simulink model "lab_5_task_2_simulink"  (R2025b)
settings: Solver=ode4  StartTime=0.0  StopTime=100  FixedStep=0.1  RelTol=1e-3
values from neighbouring files (symbols this model uses):
  I = diag([ix iy iz])    [lab_4_task_1.m]    (also in lab_5_task_1.m; lab_5_task_2.m; lab_6_task_1.m = diag([ ix iy iz ]); lab_6_task_2.m = diag([ ix iy iz ]))
  phi0 = 0    [lab_5_task_1.m]    (also in lab_5_task_2.m)
  psi0 = 0    [lab_5_task_1.m]    (also in lab_5_task_2.m)
  theta0 = 0    [lab_5_task_1.m]    (also in lab_5_task_2.m)
  w0 = [0.01 0.01 0.01]    [lab_3_task_3.m]    (also in lab_5_task_1.m = [wx0 wy0 wz0]; lab_5_task_2.m = [wx0 wy0 wz0]; lab_6_task_1.m = [wx0 wy0 wz0]; lab_6_task_2.m = [wx0 wy0 wz0])
libraries: matrix_library x2
settings Model: Creator=User  LastModifiedBy=User

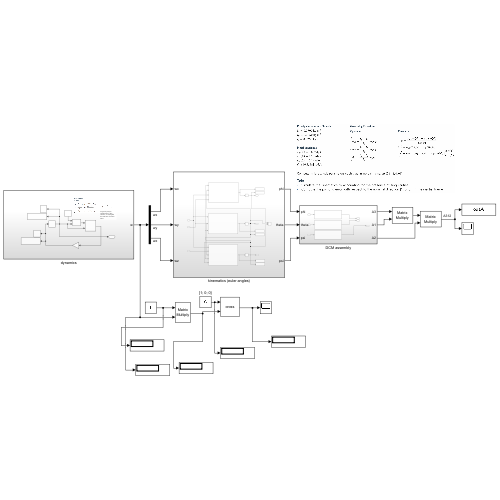
[thumbnail: Simulink's stored preview of the top-level diagram]
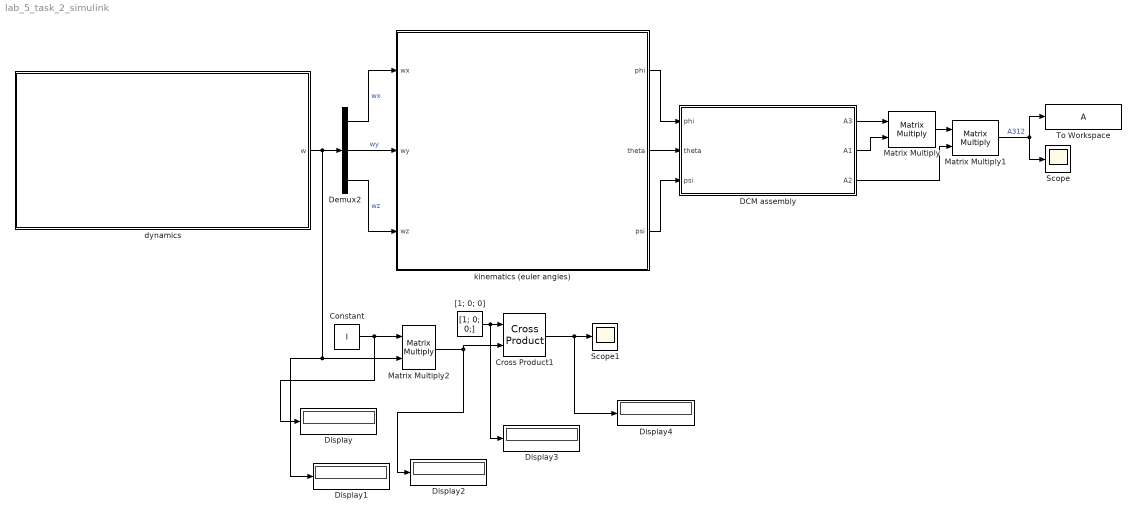
== system lab_5_task_2_simulink ==
  Constant : Constant  Value=I
  Cross Product1 : matrix_library/Cross Product
  DCM assembly : Subsystem
  Demux2 : Demux  Outputs=3
  Display{,1..4} (5 alike) : Display
  Matrix Multiply : Product  Multiplication=Matrix(*)
  Matrix Multiply1 : Product  Multiplication=Matrix(*)
  Matrix Multiply2 : Product  Multiplication=Matrix(*)
  Scope : Scope
      settings: ActiveDisplayYMinimum=-1  ActiveDisplayYMaximum=1
  Scope1 : Scope
      settings: DataLoggingVariableName=ScopeData4
  To Workspace : ToWorkspace  VariableName=A  SaveFormat=Timeseries  SampleTime=-1
  "[1; 0; 0]" : Constant  Value=[1; 0; 0;]
  dynamics : Subsystem
  kinematics (euler angles) : Subsystem
  wires:
  dynamics/1(w) -> Display1/1, Matrix Multiply2/2, Demux2/1
  DCM assembly/3(A2) -> Matrix Multiply1/2
  DCM assembly/2(A1) -> Matrix Multiply/2
  DCM assembly/1(A3) -> Matrix Multiply/1
  kinematics (euler angles)/3(psi) -> DCM assembly/3(psi)
  kinematics (euler angles)/2(theta) -> DCM assembly/2(theta)
  Demux2/2 -> kinematics (euler angles)/2(wy)  "wy"
  kinematics (euler angles)/1(phi) -> DCM assembly/1(phi)
  Demux2/3 -> kinematics (euler angles)/3(wz)  "wz"
  Matrix Multiply/1 -> Matrix Multiply1/1
  Demux2/1 -> kinematics (euler angles)/1(wx)  "wx"
  Matrix Multiply1/1 -> To Workspace/1, Scope/1  "A312"
  Constant/1 -> Display/1, Matrix Multiply2/1
  "[1; 0; 0]"/1 -> Display3/1, Cross Product1/1
  Matrix Multiply2/1 -> Display2/1, Cross Product1/2
  Cross Product1/1 -> Display4/1, Scope1/1

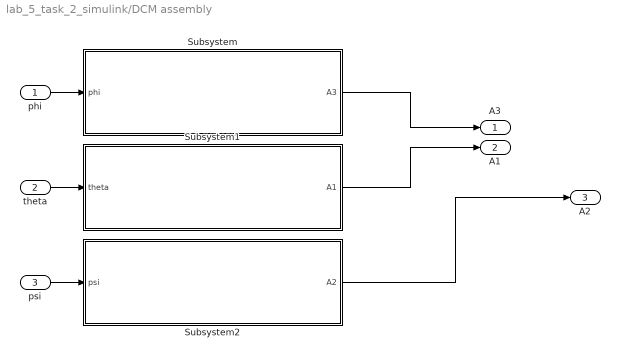
== system lab_5_task_2_simulink/DCM assembly ==
  phi : Inport
  theta : Inport  Port=2
  psi : Inport  Port=3
  Subsystem : Subsystem
  Subsystem1 : Subsystem
  Subsystem2 : Subsystem
  A3 : Outport
  A1 : Outport  Port=2
  A2 : Outport  Port=3
  wires:
  psi/1 -> Subsystem2/1(psi)
  theta/1 -> Subsystem1/1(theta)
  Subsystem1/1(A1) -> A1/1
  phi/1 -> Subsystem/1(phi)
  Subsystem/1(A3) -> A3/1
  Subsystem2/1(A2) -> A2/1

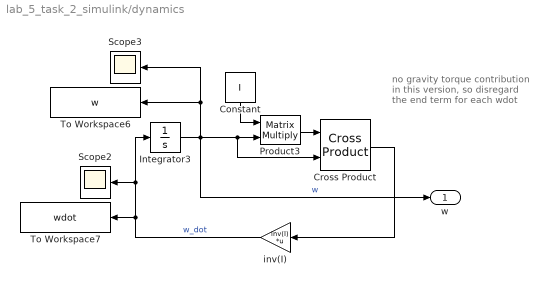
== system lab_5_task_2_simulink/dynamics ==
  note: no gravity torque contribution in this version, so disregard the end term for each wdot
  Constant : Constant  Value=I
  Cross Product : matrix_library/Cross Product
  Integrator3 : Integrator  InitialCondition=w0
  Product3 : Product  Multiplication=Matrix(*)
  Scope2 : Scope
      settings: ActiveDisplayYMinimum=-0.016616686517193405  ActiveDisplayYMaximum=0.016617993544451006  DataLoggingVariableName=ScopeData2
  Scope3 : Scope
      settings: ActiveDisplayYMinimum=-1  ActiveDisplayYMaximum=1  DataLoggingVariableName=ScopeData3
  To Workspace6 : ToWorkspace  VariableName=w  SaveFormat=Timeseries  SampleTime=-1
  To Workspace7 : ToWorkspace  VariableName=wdot  SaveFormat=Timeseries  SampleTime=-1
  inv(I) : Gain  Gain=inv(I)  Multiplication=Matrix(K*u)
  w : Outport
  wires:
  Integrator3/1 -> w/1, Cross Product/2, Product3/2, To Workspace6/1, Scope3/1  "w"
  Cross Product/1 -> inv(I)/1
  Product3/1 -> Cross Product/1
  Constant/1 -> Product3/1
  inv(I)/1 -> Scope2/1, Integrator3/1, To Workspace7/1  "w_dot"

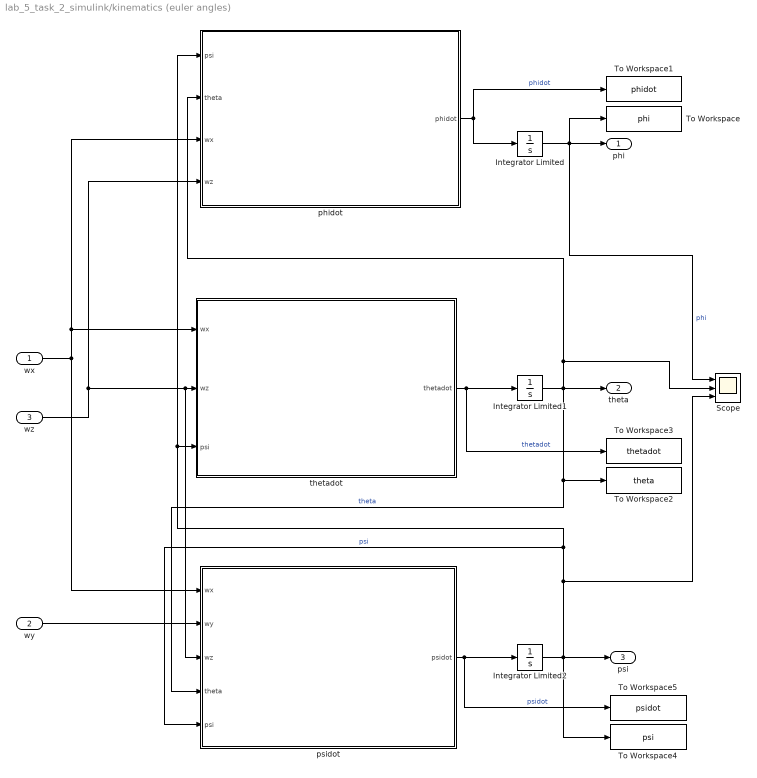
== system lab_5_task_2_simulink/kinematics (euler angles) ==
  wx : Inport
  wy : Inport  Port=2
  wz : Inport  Port=3
  Integrator Limited : Integrator  InitialCondition=phi0  LimitOutput=on  UpperSaturationLimit=2*pi  LowerSaturationLimit=0
  Integrator Limited1 : Integrator  InitialCondition=theta0  LimitOutput=on  UpperSaturationLimit=2*pi  LowerSaturationLimit=0
  Integrator Limited2 : Integrator  InitialCondition=psi0  LimitOutput=on  UpperSaturationLimit=2*pi  LowerSaturationLimit=0
  Scope : Scope  NumInputPorts=3
      settings: ActiveDisplayYMinimum=-1  ActiveDisplayYMaximum=1
  To Workspace : ToWorkspace  VariableName=phi  SaveFormat=Timeseries  SampleTime=-1
  To Workspace1 : ToWorkspace  VariableName=phidot  SaveFormat=Timeseries  SampleTime=-1
  To Workspace2 : ToWorkspace  VariableName=theta  SaveFormat=Timeseries  SampleTime=-1
  To Workspace3 : ToWorkspace  VariableName=thetadot  SaveFormat=Timeseries  SampleTime=-1
  To Workspace4 : ToWorkspace  VariableName=psi  SaveFormat=Timeseries  SampleTime=-1
  To Workspace5 : ToWorkspace  VariableName=psidot  SaveFormat=Timeseries  SampleTime=-1
  phidot : Subsystem
  psidot : Subsystem
  thetadot : Subsystem
  phi : Outport
  theta : Outport  Port=2
  psi : Outport  Port=3
  wires:
  thetadot/1(thetadot) -> Integrator Limited1/1, To Workspace3/1  "thetadot"
  Integrator Limited2/1 -> To Workspace4/1, psi/1, phidot/1(psi), thetadot/3(psi), psidot/5(psi), Scope/3  "psi"
  Integrator Limited/1 -> To Workspace/1, phi/1, Scope/1  "phi"
  wy/1 -> psidot/2(wy)
  phidot/1(phidot) -> To Workspace1/1, Integrator Limited/1  "phidot"
  wx/1 -> phidot/3(wx), thetadot/1(wx), psidot/1(wx)
  Integrator Limited1/1 -> theta/1, Scope/2, phidot/2(theta), To Workspace2/1, psidot/4(theta)  "theta"
  wz/1 -> psidot/3(wz), thetadot/2(wz), phidot/4(wz)
  psidot/1(psidot) -> To Workspace5/1, Integrator Limited2/1  "psidot"

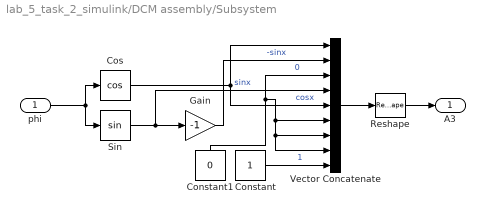
== system lab_5_task_2_simulink/DCM assembly/Subsystem ==
  phi : Inport
  Constant : Constant
  Constant1 : Constant  Value=0
  Cos : Trigonometry  Operator=cos
  Gain : Gain  Gain=-1
  Reshape : Reshape  OutputDimensionality=Customize  OutputDimensions=[3,3]
  Sin : Trigonometry
  Vector Concatenate : Concatenate  NumInputs=9
  A3 : Outport
  wires:
  Constant/1 -> Vector Concatenate/9  "1"
  Gain/1 -> Vector Concatenate/2  "-sinx"
  Sin/1 -> Vector Concatenate/4, Gain/1  "sinx"
  Constant1/1 -> Vector Concatenate/8, Vector Concatenate/7, Vector Concatenate/6, Vector Concatenate/3  "0"
  Cos/1 -> Vector Concatenate/1, Vector Concatenate/5  "cosx"
  phi/1 -> Sin/1, Cos/1
  Vector Concatenate/1 -> Reshape/1
  Reshape/1 -> A3/1

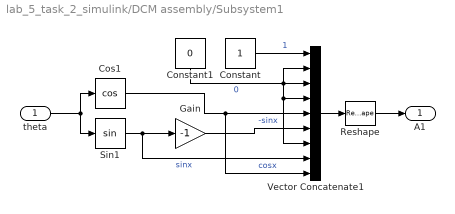
== system lab_5_task_2_simulink/DCM assembly/Subsystem1 ==
  theta : Inport
  Constant : Constant
  Constant1 : Constant  Value=0
  Cos1 : Trigonometry  Operator=cos
  Gain : Gain  Gain=-1
  Reshape : Reshape  OutputDimensionality=Customize  OutputDimensions=[3,3]
  Sin1 : Trigonometry
  Vector Concatenate1 : Concatenate  NumInputs=9
  A1 : Outport
  wires:
  theta/1 -> Sin1/1, Cos1/1
  Constant1/1 -> Vector Concatenate1/7, Vector Concatenate1/4, Vector Concatenate1/3, Vector Concatenate1/2  "0"
  Cos1/1 -> Vector Concatenate1/9, Vector Concatenate1/5  "cosx"
  Gain/1 -> Vector Concatenate1/6  "-sinx"
  Sin1/1 -> Vector Concatenate1/8, Gain/1  "sinx"
  Constant/1 -> Vector Concatenate1/1  "1"
  Vector Concatenate1/1 -> Reshape/1
  Reshape/1 -> A1/1

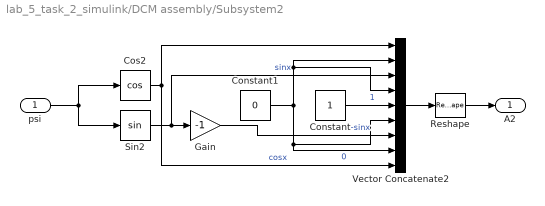
== system lab_5_task_2_simulink/DCM assembly/Subsystem2 ==
  psi : Inport
  Constant : Constant
  Constant1 : Constant  Value=0
  Cos2 : Trigonometry  Operator=cos
  Gain : Gain  Gain=-1
  Reshape : Reshape  OutputDimensionality=Customize  OutputDimensions=[3,3]
  Sin2 : Trigonometry
  Vector Concatenate2 : Concatenate  NumInputs=9
  A2 : Outport
  wires:
  Sin2/1 -> Vector Concatenate2/3, Gain/1  "sinx"
  Constant/1 -> Vector Concatenate2/5  "1"
  Constant1/1 -> Vector Concatenate2/8, Vector Concatenate2/6, Vector Concatenate2/4, Vector Concatenate2/2  "0"
  Vector Concatenate2/1 -> Reshape/1
  Gain/1 -> Vector Concatenate2/7  "-sinx"
  Cos2/1 -> Vector Concatenate2/9, Vector Concatenate2/1  "cosx"
  psi/1 -> Sin2/1, Cos2/1
  Reshape/1 -> A2/1

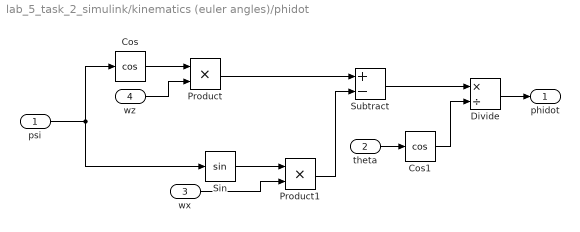
== system lab_5_task_2_simulink/kinematics (euler angles)/phidot ==
  psi : Inport
  theta : Inport  Port=2
  wx : Inport  Port=3
  wz : Inport  Port=4
  Cos : Trigonometry  Operator=cos
  Cos1 : Trigonometry  Operator=cos
  Divide : Product  Inputs=*/
  Product : Product
  Product1 : Product
  Sin : Trigonometry
  Subtract : Sum  Inputs=+-
  phidot : Outport
  wires:
  Sin/1 -> Product1/1
  Subtract/1 -> Divide/1
  Divide/1 -> phidot/1
  psi/1 -> Sin/1, Cos/1
  Cos/1 -> Product/1
  theta/1 -> Cos1/1
  Product/1 -> Subtract/1
  Cos1/1 -> Divide/2
  Product1/1 -> Subtract/2
  wx/1 -> Product1/2
  wz/1 -> Product/2

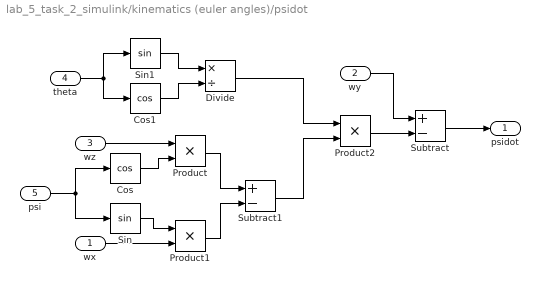
== system lab_5_task_2_simulink/kinematics (euler angles)/psidot ==
  wx : Inport
  wy : Inport  Port=2
  wz : Inport  Port=3
  theta : Inport  Port=4
  psi : Inport  Port=5
  Cos : Trigonometry  Operator=cos
  Cos1 : Trigonometry  Operator=cos
  Divide : Product  Inputs=*/
  Product : Product
  Product1 : Product
  Product2 : Product
  Sin : Trigonometry
  Sin1 : Trigonometry
  Subtract : Sum  Inputs=+-
  Subtract1 : Sum  Inputs=+-
  psidot : Outport
  wires:
  Product1/1 -> Subtract1/2
  Subtract1/1 -> Product2/2
  wy/1 -> Subtract/1
  Sin1/1 -> Divide/1
  Cos1/1 -> Divide/2
  Divide/1 -> Product2/1
  Subtract/1 -> psidot/1
  theta/1 -> Sin1/1, Cos1/1
  Cos/1 -> Product/2
  psi/1 -> Sin/1, Cos/1
  Product/1 -> Subtract1/1
  Product2/1 -> Subtract/2
  Sin/1 -> Product1/1
  wz/1 -> Product/1
  wx/1 -> Product1/2

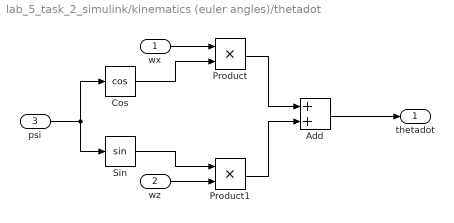
== system lab_5_task_2_simulink/kinematics (euler angles)/thetadot ==
  wx : Inport
  wz : Inport  Port=2
  psi : Inport  Port=3
  Add : Sum
  Cos : Trigonometry  Operator=cos
  Product : Product
  Product1 : Product
  Sin : Trigonometry
  thetadot : Outport
  wires:
  Add/1 -> thetadot/1
  wx/1 -> Product/1
  Product1/1 -> Add/2
  psi/1 -> Sin/1, Cos/1
  Product/1 -> Add/1
  wz/1 -> Product1/2
  Cos/1 -> Product/2
  Sin/1 -> Product1/1
